simulink model "Cruise_Model_V8_QRTuning_TFLim"  (R2024a)
settings: Solver=ode23t  StartTime=0.0  StopTime=20  RelTol=1e-3
values from neighbouring files (symbols this model uses):
  F = fullfile(P,S(k).name)    [extractNACAdata.m]
  mission = struct()    [runMission.m]
  r = fuselage(i).diameter/2    [plotConfiguration.m]
  referenceGeo =     [alexisignoringme.mat]    (also in testing.mat)
undefined symbols (not defined in the file or in its folder): coefficients, dir, K, kb, kt, Light, MIL, Ue, Xe, Xes, xyz_tr
libraries: slpidlib x14, aerolibwind2 x8, aerolibatmos2 x4, shared6dof x1
(part 2 of 3)

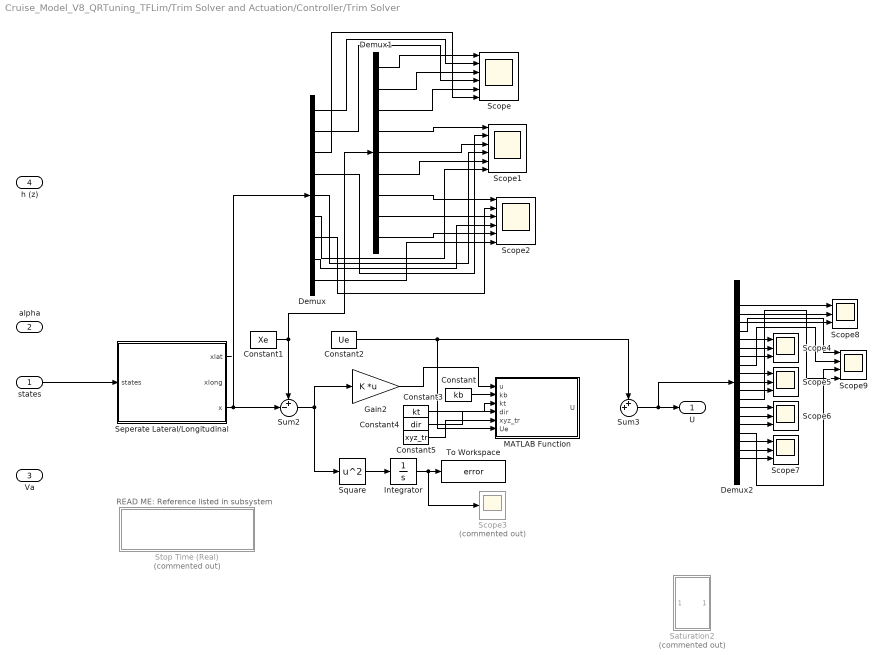
== system Cruise_Model_V8_QRTuning_TFLim/Trim Solver and Actuation/Controller/Trim Solver ==
  note: READ ME: Reference listed in subsystem
  states : Inport
  alpha : Inport  Port=2
  Va : Inport  Port=3
  h (z) : Inport  Port=4
  Constant : Constant  Value=kb
  Constant1 : Constant  Value=Xe
  Constant2 : Constant  Value=Ue
  Constant3 : Constant  Value=kt
  Constant4 : Constant  Value=dir
  Constant5 : Constant  Value=xyz_tr
  Demux : Demux  Outputs=9
  Demux1 : Demux  Outputs=9
  Demux2 : Demux  Outputs=19
  Gain2 : Gain  Gain=K  Multiplication=Matrix(K*u) (u vector)
  Integrator : Integrator
  MATLAB Function : MATLAB Function  TreatAsAtomicUnit=on
  Saturation2 : Subsystem  Commented=on
  Scope : Scope  NumInputPorts=6
  Scope1 : Scope  NumInputPorts=6
  Scope2 : Scope  NumInputPorts=6
  Scope3 : Scope  Commented=on
  Scope{4..8} (5 alike) : Scope  NumInputPorts=3
  Scope9 : Scope  NumInputPorts=4
  Seperate Lateral/Longitudinal : Subsystem
  Square : Math  Operator=square
  Stop Time (Real) : Subsystem  Commented=on
  Sum2 : Sum  Inputs=+-|
  Sum3 : Sum  Inputs=++|
  To Workspace : ToWorkspace  VariableName=error  SaveFormat=Timeseries  SampleTime=-1
  U : Outport
  wires:
  states/1 -> Seperate Lateral/Longitudinal/1(states)
  Seperate Lateral/Longitudinal/1(xlat) -> ?
  Seperate Lateral/Longitudinal/3(x) -> Demux/1, Sum2/2
  Constant2/1 -> Sum3/1, MATLAB Function/6(Ue)
  Constant1/1 -> Sum2/1, Demux1/1
  Square/1 -> Integrator/1
  Sum2/1 -> Square/1, Gain2/1
  Integrator/1 -> Scope3/1, To Workspace/1
  Demux1/1 -> Scope/1
  Demux/1 -> Scope/2
  Demux1/2 -> Scope/3
  Demux/2 -> Scope/4
  Demux1/3 -> Scope/5
  Demux/3 -> Scope/6
  Demux1/4 -> Scope1/1
  Demux1/5 -> Scope1/3
  Demux1/6 -> Scope1/5
  Demux/4 -> Scope1/2
  Demux/5 -> Scope1/4
  Demux/6 -> Scope1/6
  Demux1/7 -> Scope2/1
  Demux1/8 -> Scope2/3
  Demux1/9 -> Scope2/5
  Demux/7 -> Scope2/2
  Demux/8 -> Scope2/4
  Demux/9 -> Scope2/6
  Demux2/5 -> Scope4/1
  Demux2/6 -> Scope4/2
  Demux2/7 -> Scope4/3
  Demux2/9 -> Scope5/1
  Demux2/10 -> Scope5/2
  Demux2/11 -> Scope5/3
  Demux2/13 -> Scope6/1
  Demux2/14 -> Scope6/2
  Demux2/15 -> Scope6/3
  Demux2/17 -> Scope7/1
  Demux2/18 -> Scope7/2
  Demux2/19 -> Scope7/3
  Sum3/1 -> U/1, Demux2/1
  Gain2/1 -> MATLAB Function/1(u)
  Demux2/1 -> Scope8/1
  Demux2/2 -> Scope8/2
  Demux2/3 -> Scope8/3
  Demux2/4 -> Scope9/1
  Demux2/8 -> Scope9/2
  Demux2/12 -> Scope9/4
  Demux2/16 -> Scope9/3
  Constant/1 -> MATLAB Function/2(kb)
  Constant3/1 -> MATLAB Function/3(kt)
  Constant4/1 -> MATLAB Function/4(dir)
  Constant5/1 -> MATLAB Function/5(xyz_tr)

== system Cruise_Model_V8_QRTuning_TFLim/Atmospheric Effects/Atmospheric Effects1/Variant Subsystem/a ==
  h (z) : Inport
  Constant : Constant  Value=0
  ISA Atmosphere : aerolibatmos2/ISA Atmosphere Model  useExtended=off  action=Warning  custom=off  viscosityOut=off  g=9.80665  gamma=1.4  R=287.0531  L=0.0065  h_trop=11000  h_strat=20000  rho0=1.225  P0=101325  T0=288.15  h0=0  S=110.4  Tref=273.15  muref=1.716e-5
  Terminator1 : Terminator
  Terminator2 : Terminator
  Terminator3 : Terminator
  Air Density : Outport
  Vw : Outport  Port=2
  wires:
  h (z)/1 -> ISA Atmosphere/1
  ISA Atmosphere/2 -> Terminator1/1
  ISA Atmosphere/1 -> Terminator3/1
  ISA Atmosphere/4 -> Air Density/1
  ISA Atmosphere/3 -> Terminator2/1
  Constant/1 -> Vw/1

== system Cruise_Model_V8_QRTuning_TFLim/Atmospheric Effects/Atmospheric Effects1/Variant Subsystem/ag ==
  uvw_e : Inport
  h (z) : Inport  Port=2
  Demux : Demux  Outputs=3
  Discrete Wind Gust Model : aerolibwind2/Discrete Wind Gust Model  units=Metric (MKS)  Gx=on  Gy=on  Gz=on  t_0=40  d_m=[120 120 80]  v_m=[10 10 10]
  ISA Atmosphere : aerolibatmos2/ISA Atmosphere Model  useExtended=off  action=Warning  custom=off  viscosityOut=off  g=9.80665  gamma=1.4  R=287.0531  L=0.0065  h_trop=11000  h_strat=20000  rho0=1.225  P0=101325  T0=288.15  h0=0  S=110.4  Tref=273.15  muref=1.716e-5
  Terminator1 : Terminator
  Terminator2 : Terminator
  Terminator3 : Terminator
  Vw : Outport
  Air Density : Outport  Port=2
  wires:
  h (z)/1 -> ISA Atmosphere/1
  Demux/1 -> Discrete Wind Gust Model/1
  ISA Atmosphere/2 -> Terminator1/1
  ISA Atmosphere/1 -> Terminator3/1
  ISA Atmosphere/4 -> Air Density/1
  uvw_e/1 -> Demux/1
  ISA Atmosphere/3 -> Terminator2/1
  Discrete Wind Gust Model/1 -> Vw/1

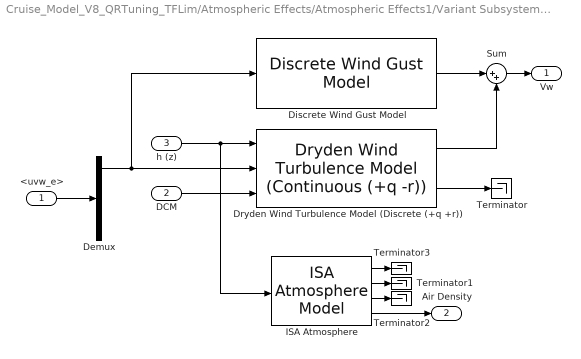
== system Cruise_Model_V8_QRTuning_TFLim/Atmospheric Effects/Atmospheric Effects1/Variant Subsystem/agt ==
  <uvw_e> : Inport
  DCM : Inport  Port=2
  h (z) : Inport  Port=3
  Demux : Demux  Outputs=3
  Discrete Wind Gust Model : aerolibwind2/Discrete Wind Gust Model  units=Metric (MKS)  Gx=on  Gy=on  Gz=on  t_0=40  d_m=[120 120 80]  v_m=[10 10 10]
  Dryden Wind Turbulence Model (Discrete (+q +r)) : aerolibwind2/Dryden Wind Turbulence Model  (Continuous (+q -r))  units=Metric (MKS)  spec=MIL-F-8785C  model=Continuous Dryden (+q -r)  W20=10  Wdeg=8  TurbProb=10^-2 - Light  L_high=533.4  Wingspan=7  ts=0.1  Seed=[23341 23342 23343 23344]  T_on=on
      settings: LibrarySourceBlock=|
      | aerolibwind2/Dryden Wind Turbulence Model
      | (Discrete (+q +r))
  ISA Atmosphere : aerolibatmos2/ISA Atmosphere Model  useExtended=off  action=Warning  custom=off  viscosityOut=off  g=9.80665  gamma=1.4  R=287.0531  L=0.0065  h_trop=11000  h_strat=20000  rho0=1.225  P0=101325  T0=288.15  h0=0  S=110.4  Tref=273.15  muref=1.716e-5
  Sum : Sum  Inputs=|++
  Terminator{,1..3} (4 alike) : Terminator
  Vw : Outport
  Air Density : Outport  Port=2
  wires:
  h (z)/1 -> Dryden Wind Turbulence Model (Discrete (+q +r))/1, ISA Atmosphere/1
  Demux/1 -> Dryden Wind Turbulence Model (Discrete (+q +r))/2, Discrete Wind Gust Model/1
  ISA Atmosphere/2 -> Terminator1/1
  ISA Atmosphere/1 -> Terminator3/1
  ISA Atmosphere/4 -> Air Density/1
  <uvw_e>/1 -> Demux/1
  DCM/1 -> Dryden Wind Turbulence Model (Discrete (+q +r))/3
  Dryden Wind Turbulence Model (Discrete (+q +r))/2 -> Terminator/1
  Sum/1 -> Vw/1
  ISA Atmosphere/3 -> Terminator2/1
  Dryden Wind Turbulence Model (Discrete (+q +r))/1 -> Sum/2
  Discrete Wind Gust Model/1 -> Sum/1

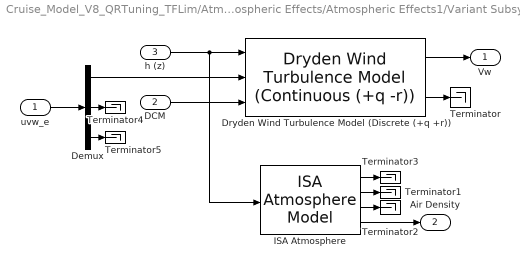
== system Cruise_Model_V8_QRTuning_TFLim/Atmospheric Effects/Atmospheric Effects1/Variant Subsystem/at ==
  uvw_e : Inport
  DCM : Inport  Port=2
  h (z) : Inport  Port=3
  Demux : Demux  Outputs=3
  Dryden Wind Turbulence Model (Discrete (+q +r)) : aerolibwind2/Dryden Wind Turbulence Model  (Continuous (+q -r))  units=Metric (MKS)  spec=MIL-F-8785C  model=Continuous Dryden (+q -r)  W20=10  Wdeg=8  TurbProb=10^-2 - Light  L_high=533.4  Wingspan=7  ts=0.1  Seed=[23341 23342 23343 23344]  T_on=on
      settings: LibrarySourceBlock=|
      | aerolibwind2/Dryden Wind Turbulence Model
      | (Discrete (+q +r))
  ISA Atmosphere : aerolibatmos2/ISA Atmosphere Model  useExtended=off  action=Warning  custom=off  viscosityOut=off  g=9.80665  gamma=1.4  R=287.0531  L=0.0065  h_trop=11000  h_strat=20000  rho0=1.225  P0=101325  T0=288.15  h0=0  S=110.4  Tref=273.15  muref=1.716e-5
  Terminator{,1..5} (6 alike) : Terminator
  Vw : Outport
  Air Density : Outport  Port=2
  wires:
  h (z)/1 -> Dryden Wind Turbulence Model (Discrete (+q +r))/1, ISA Atmosphere/1
  Demux/1 -> Dryden Wind Turbulence Model (Discrete (+q +r))/2
  ISA Atmosphere/2 -> Terminator1/1
  ISA Atmosphere/1 -> Terminator3/1
  ISA Atmosphere/4 -> Air Density/1
  uvw_e/1 -> Demux/1
  DCM/1 -> Dryden Wind Turbulence Model (Discrete (+q +r))/3
  Dryden Wind Turbulence Model (Discrete (+q +r))/2 -> Terminator/1
  ISA Atmosphere/3 -> Terminator2/1
  Demux/2 -> Terminator4/1
  Demux/3 -> Terminator5/1
  Dryden Wind Turbulence Model (Discrete (+q +r))/1 -> Vw/1

== system Cruise_Model_V8_QRTuning_TFLim/Atmospheric Effects/Atmospheric Effects1/Variant Subsystem/g ==
  uvw_e : Inport
  Constant : Constant  Value=1.225
  Demux : Demux  Outputs=3
  Discrete Wind Gust Model : aerolibwind2/Discrete Wind Gust Model  units=Metric (MKS)  Gx=on  Gy=on  Gz=on  t_0=40  d_m=[120 120 80]  v_m=[10 10 10]
  Vw : Outport
  Air Density : Outport  Port=2
  wires:
  Demux/1 -> Discrete Wind Gust Model/1
  uvw_e/1 -> Demux/1
  Discrete Wind Gust Model/1 -> Vw/1
  Constant/1 -> Air Density/1

== system Cruise_Model_V8_QRTuning_TFLim/Atmospheric Effects/Atmospheric Effects1/Variant Subsystem/gt ==
  <uvw_e> : Inport
  DCM : Inport  Port=2
  h (z) : Inport  Port=3
  Constant : Constant  Value=1.225
  Demux : Demux  Outputs=3
  Discrete Wind Gust Model : aerolibwind2/Discrete Wind Gust Model  units=Metric (MKS)  Gx=on  Gy=on  Gz=on  t_0=40  d_m=[120 120 80]  v_m=[10 10 10]
  Dryden Wind Turbulence Model (Discrete (+q +r)) : aerolibwind2/Dryden Wind Turbulence Model  (Continuous (+q -r))  units=Metric (MKS)  spec=MIL-F-8785C  model=Continuous Dryden (+q -r)  W20=10  Wdeg=8  TurbProb=10^-2 - Light  L_high=533.4  Wingspan=7  ts=0.1  Seed=[23341 23342 23343 23344]  T_on=on
      settings: LibrarySourceBlock=|
      | aerolibwind2/Dryden Wind Turbulence Model
      | (Discrete (+q +r))
  Sum : Sum  Inputs=|++
  Terminator : Terminator
  Vw : Outport
  Air Density : Outport  Port=2
  wires:
  h (z)/1 -> Dryden Wind Turbulence Model (Discrete (+q +r))/1
  Demux/1 -> Dryden Wind Turbulence Model (Discrete (+q +r))/2, Discrete Wind Gust Model/1
  <uvw_e>/1 -> Demux/1
  DCM/1 -> Dryden Wind Turbulence Model (Discrete (+q +r))/3
  Dryden Wind Turbulence Model (Discrete (+q +r))/2 -> Terminator/1
  Sum/1 -> Vw/1
  Dryden Wind Turbulence Model (Discrete (+q +r))/1 -> Sum/2
  Discrete Wind Gust Model/1 -> Sum/1
  Constant/1 -> Air Density/1

== system Cruise_Model_V8_QRTuning_TFLim/Atmospheric Effects/Atmospheric Effects1/Variant Subsystem/n ==
  Constant : Constant  Value=0
  Constant1 : Constant  Value=1.225
  Vw : Outport
  Air Density : Outport  Port=2
  wires:
  Constant/1 -> Vw/1
  Constant1/1 -> Air Density/1

== system Cruise_Model_V8_QRTuning_TFLim/Atmospheric Effects/Atmospheric Effects1/Variant Subsystem/t ==
  <uvw_e> : Inport
  DCM : Inport  Port=2
  h (z) : Inport  Port=3
  Constant1 : Constant  Value=1.225
  Demux : Demux  Outputs=3
  Dryden Wind Turbulence Model (Discrete (+q +r)) : aerolibwind2/Dryden Wind Turbulence Model  (Continuous (+q -r))  units=Metric (MKS)  spec=MIL-F-8785C  model=Continuous Dryden (+q -r)  W20=10  Wdeg=8  TurbProb=10^-2 - Light  L_high=533.4  Wingspan=7  ts=0.1  Seed=[23341 23342 23343 23344]  T_on=on
      settings: LibrarySourceBlock=|
      | aerolibwind2/Dryden Wind Turbulence Model
      | (Discrete (+q +r))
  Terminator : Terminator
  Vw : Outport
  Air Density : Outport  Port=2
  wires:
  h (z)/1 -> Dryden Wind Turbulence Model (Discrete (+q +r))/1
  Demux/1 -> Dryden Wind Turbulence Model (Discrete (+q +r))/2
  <uvw_e>/1 -> Demux/1
  DCM/1 -> Dryden Wind Turbulence Model (Discrete (+q +r))/3
  Dryden Wind Turbulence Model (Discrete (+q +r))/2 -> Terminator/1
  Constant1/1 -> Air Density/1
  Dryden Wind Turbulence Model (Discrete (+q +r))/1 -> Vw/1

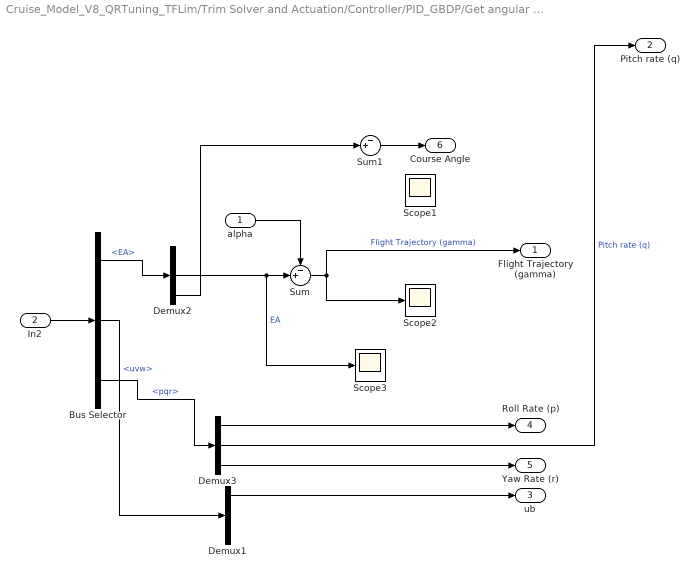
== system Cruise_Model_V8_QRTuning_TFLim/Trim Solver and Actuation/Controller/PID_GBDP/Get angular properties ==
  alpha : Inport
  In2 : Inport  Port=2
  Bus Selector : BusSelector  OutputSignals=EA,uvw,pqr
  Demux1 : Demux  Outputs=3
  Demux2 : Demux  Outputs=3
  Demux3 : Demux  Outputs=3
  Scope1 : Scope
  Scope2 : Scope
  Scope3 : Scope
  Sum : Sum  Inputs=-+|
  Sum1 : Sum  Inputs=-+|
  Flight Trajectory (gamma) : Outport
  Pitch rate (q) : Outport  Port=2
  ub : Outport  Port=3
  Roll Rate (p) : Outport  Port=4
  Yaw Rate (r) : Outport  Port=5
  Course Angle : Outport  Port=6
  wires:
  alpha/1 -> Sum/1
  Demux2/2 -> Sum/2, Scope3/1  "EA"
  Bus Selector/3 -> Demux3/1  "<pqr>"
  Sum/1 -> Flight Trajectory (gamma)/1, Scope2/1  "Flight Trajectory (gamma)"
  Bus Selector/1 -> Demux2/1  "<EA>"
  In2/1 -> Bus Selector/1
  Demux3/2 -> Pitch rate (q)/1  "Pitch rate (q)"
  Bus Selector/2 -> Demux1/1  "<uvw>"
  Demux1/1 -> ub/1
  Demux3/1 -> Roll Rate (p)/1
  Sum1/1 -> Course Angle/1
  Demux3/3 -> Yaw Rate (r)/1
  Demux2/3 -> Sum1/2

== system Cruise_Model_V8_QRTuning_TFLim/Trim Solver and Actuation/Controller/PID_GBDP/Step demand for testing ==
  In1 : Inport
  Mux1 : Mux  Inputs=2
  Scope2 : Scope
  Scope4 : Scope
  Step1 : Step  Time=60  Before=-500  After=-490  SampleTime=0
  Step2 : Step  Time=80  After=-10  SampleTime=0
  Step3 : Step  Time=120  After=20  SampleTime=0
  Step4 : Step  Time=120  After=20  SampleTime=0
  Sum : Sum  Inputs=++++
  To Workspace : ToWorkspace  VariableName=altitudeResponse  SaveFormat=Timeseries  SampleTime=-1
  Out1 : Outport
  wires:
  Step3/1 -> Sum/3
  Mux1/1 -> To Workspace/1, Scope4/1
  Sum/1 -> Out1/1, Mux1/1
  Step4/1 -> Sum/4
  Step1/1 -> Sum/1
  In1/1 -> Mux1/2, Scope2/1
  Step2/1 -> Sum/2

== system Cruise_Model_V8_QRTuning_TFLim/Trim Solver and Actuation/Controller/PID_GBDP/Step demand for testing1 ==
  Va : Inport
  Mux1 : Mux  Inputs=2
  Scope2 : Scope
  Scope4 : Scope
  Step1 : Step  Time=60  Before=25  After=31  SampleTime=0
  Step2 : Step  Time=80  After=-3  SampleTime=0
  Step3 : Step  Time=120  After=-5  SampleTime=0
  Step4 : Step  Time=100  After=8  SampleTime=0
  Step5 : Step  Time=140  After=-2  SampleTime=0
  Sum : Sum  Inputs=+++++
  To Workspace : ToWorkspace  VariableName=airspeedResponse  SaveFormat=Timeseries  SampleTime=-1
  Out1 : Outport
  wires:
  Step2/1 -> Sum/2
  Va/1 -> Scope2/1, Mux1/2
  Step1/1 -> Sum/1
  Step4/1 -> Sum/4
  Sum/1 -> Mux1/1, Out1/1
  Mux1/1 -> Scope4/1, To Workspace/1
  Step3/1 -> Sum/3
  Step5/1 -> Sum/5

== system Cruise_Model_V8_QRTuning_TFLim/Trim Solver and Actuation/Controller/PID_GBDP/Step demand for testing2 ==
  Va : Inport
  Mux1 : Mux  Inputs=2
  Scope2 : Scope
  Scope4 : Scope
  Step1 : Step  Time=60  Before=0.1  After=0.2  SampleTime=0
  Step2 : Step  Time=80  After=-0.4  SampleTime=0
  Step3 : Step  Time=120  After=-0.2  SampleTime=0
  Step4 : Step  Time=100  After=0.6  SampleTime=0
  Step5 : Step  Time=140  After=-0.4  SampleTime=0
  Sum : Sum  Inputs=+++++
  To Workspace : ToWorkspace  VariableName=headingAngleResponse  SaveFormat=Timeseries  SampleTime=-1
  Out1 : Outport
  wires:
  Step5/1 -> Sum/5
  Step3/1 -> Sum/3
  Mux1/1 -> To Workspace/1, Scope4/1
  Sum/1 -> Out1/1, Mux1/1
  Step4/1 -> Sum/4
  Step1/1 -> Sum/1
  Va/1 -> Mux1/2, Scope2/1
  Step2/1 -> Sum/2

== system Cruise_Model_V8_QRTuning_TFLim/Trim Solver and Actuation/Controller/PID_GBDP_withThrust/Altitude Control Path ==
  note: Altitude Control Path
  h (z) : Inport
  Flight Trajectory : Inport  Port=2
  Pitch Rate : Inport  Port=3
  Demand : Inport  Port=4
  PID Controller10 : slpidlib/PID Controller  Controller=PID  Form=Parallel  TimeDomain=Continuous-time  UseExternalTs=off  SampleTime=-1  IntegratorMethod=Forward Euler  FilterMethod=Forward Euler  ControllerParametersSource=internal  P=-0.89713711901533  I=-27.659938076894  UseKiTs=off  D=-0.00302643608728309  UseExternalDerivativeSource=off  N=142.832860389355  UseFilter=on  TunerSelectOption=Transfer Function Based (PID Tuner App)  InitialConditionSource=internal  InitialConditionForIntegrator=0.44  InitialConditionForFilter=0  DifferentiatorICPrevScaledInput=0  ExternalReset=none  TrackingMode=off  Kt=1  LimitOutput=on  SatLimitsSource=internal  UpperSaturationLimit=0.44  LowerSaturationLimit=-0.44  LinearizeAsGain=on  AntiWindupMode=clamping  Kb=1  LimitIntegrator=off  UpperIntegratorSaturationLimit=inf  LowerIntegratorSaturationLimit=-inf  POutMin=[]  POutMax=[]  IOutMin=[]  IOutMax=[]  DOutMin=[]  DOutMax=[]  NOutMin=[]  NOutMax=[]  SumOutMin=[]  SumOutMax=[]  SaturationOutMin=[]  SaturationOutMax=[]  PParamMin=[]  PParamMax=[]  IParamMin=[]  IParamMax=[]  DParamMin=[]  DParamMax=[]  NParamMin=[]  NParamMax=[]  KbParamMin=[]  KbParamMax=[]  KtParamMin=[]  KtParamMax=[]  KbOutMin=[]  KbOutMax=[]  KtOutMin=[]  KtOutMax=[]  IntegratorOutMin=[]  IntegratorOutMax=[]  FilterOutMin=[]  FilterOutMax=[]  SumI1OutMin=[]  SumI1OutMax=[]  SumI2OutMin=[]  SumI2OutMax=[]  SumI3OutMin=[]  SumI3OutMax=[]  SumI4OutMin=[]  SumI4OutMax=[]  SumDOutMin=[]  SumDOutMax=[]  DifferentiatorOutMin=[]  DifferentiatorOutMax=[]  FilterDiffOutCoefMin=[]  FilterDiffOutCoefMax=[]  ReciprocalOutMin=[]  ReciprocalOutMax=[]  SumDenOutMin=[]  SumDenOutMax=[]  SumNumOutMin=[]  SumNumOutMax=[]  DivideOutMin=[]  DivideOutMax=[]  UdiffTsProdOutMin=[]  UdiffTsProdOutMax=[]  NTsProdOutMin=[]  NTsProdOutMax=[]  UintegralTsProdOutMin=[]  UintegralTsProdOutMax=[]  UngainTsProdOutMin=[]  UngainTsProdOutMax=[]  ClampingZeroOutDataTypeStr=Inherit: Inherit via back propagation  ClampingZeroOutMin=[]  ClampingZeroOutMax=[]  FilterDenConstantOutDataTypeStr=Inherit: Inherit via back propagation  FilterDenConstantOutMin=[]  FilterDenConstantOutMax=[]  PCopyOutDataTypeStr=Inherit: Inherit via back propagation  PCopyOutMin=[]  PCopyOutMax=[]  NCopyOutDataTypeStr=Inherit: Inherit via back propagation  NCopyOutMin=[]  NCopyOutMax=[]  IntegratorContinuousStateAttributes=''  IntegratorStateMustResolveToSignalObject=off  IntegratorRTWStateStorageClass=Auto  FilterContinuousStateAttributes=''  FilterStateMustResolveToSignalObject=off  FilterRTWStateStorageClass=Auto  ParallelPVariant=InternalParameters  IdealPVariant=Disabled  IVariant=InternalParameters  DVariant=InternalParameters  IntegratorVariant=Continuous  SatVariant=Enabled  AWVariant=ContClampingParallel  PCopyVariant=Disabled  TRVariant=Disabled  FdbkBlocksVariant=Forward  IdealPFdbkVariant=Disabled  SatFdbkVariant=Disabled  DerivativeFilterVariant=ContFilter  NVariant=InternalParameters  NCopyVariant=Disabled  FilterICVariant=InternalICsFilter  IntegratorICVariant=InternalICs  ExternalResetVariant=Disabled  TRSumVariant=Passthrough  SumFdbkVariant=Disabled  SumVariant=Sum_PID  TsampFilterVariant=InternalTs  TsampNgainVariant=Passthrough  TsampIntegralVariant=Disabled_SignalSpec  ExternalSaturationOutDataTypeStr=Inherit: Same as second input  DerivativeSourceVariant=ErrorSignal
  PID Controller4 : slpidlib/PID Controller  Controller=PID  Form=Parallel  TimeDomain=Continuous-time  UseExternalTs=off  SampleTime=-1  IntegratorMethod=Forward Euler  FilterMethod=Forward Euler  ControllerParametersSource=internal  P=-0.487630187489664  I=-0.0704619791070383  UseKiTs=off  D=-0.813392530162756  UseExternalDerivativeSource=off  N=7.99704030727873  UseFilter=on  TunerSelectOption=Transfer Function Based (PID Tuner App)  InitialConditionSource=internal  InitialConditionForIntegrator=0.1  InitialConditionForFilter=0  DifferentiatorICPrevScaledInput=0  ExternalReset=none  TrackingMode=off  Kt=1  LimitOutput=on  SatLimitsSource=internal  UpperSaturationLimit=0.44  LowerSaturationLimit=-0.44  LinearizeAsGain=on  AntiWindupMode=clamping  Kb=1  LimitIntegrator=off  UpperIntegratorSaturationLimit=inf  LowerIntegratorSaturationLimit=-inf  POutMin=[]  POutMax=[]  IOutMin=[]  IOutMax=[]  DOutMin=[]  DOutMax=[]  NOutMin=[]  NOutMax=[]  SumOutMin=[]  SumOutMax=[]  SaturationOutMin=[]  SaturationOutMax=[]  PParamMin=[]  PParamMax=[]  IParamMin=[]  IParamMax=[]  DParamMin=[]  DParamMax=[]  NParamMin=[]  NParamMax=[]  KbParamMin=[]  KbParamMax=[]  KtParamMin=[]  KtParamMax=[]  KbOutMin=[]  KbOutMax=[]  KtOutMin=[]  KtOutMax=[]  IntegratorOutMin=[]  IntegratorOutMax=[]  FilterOutMin=[]  FilterOutMax=[]  SumI1OutMin=[]  SumI1OutMax=[]  SumI2OutMin=[]  SumI2OutMax=[]  SumI3OutMin=[]  SumI3OutMax=[]  SumI4OutMin=[]  SumI4OutMax=[]  SumDOutMin=[]  SumDOutMax=[]  DifferentiatorOutMin=[]  DifferentiatorOutMax=[]  FilterDiffOutCoefMin=[]  FilterDiffOutCoefMax=[]  ReciprocalOutMin=[]  ReciprocalOutMax=[]  SumDenOutMin=[]  SumDenOutMax=[]  SumNumOutMin=[]  SumNumOutMax=[]  DivideOutMin=[]  DivideOutMax=[]  UdiffTsProdOutMin=[]  UdiffTsProdOutMax=[]  NTsProdOutMin=[]  NTsProdOutMax=[]  UintegralTsProdOutMin=[]  UintegralTsProdOutMax=[]  UngainTsProdOutMin=[]  UngainTsProdOutMax=[]  ClampingZeroOutDataTypeStr=Inherit: Inherit via back propagation  ClampingZeroOutMin=[]  ClampingZeroOutMax=[]  FilterDenConstantOutDataTypeStr=Inherit: Inherit via back propagation  FilterDenConstantOutMin=[]  FilterDenConstantOutMax=[]  PCopyOutDataTypeStr=Inherit: Inherit via back propagation  PCopyOutMin=[]  PCopyOutMax=[]  NCopyOutDataTypeStr=Inherit: Inherit via back propagation  NCopyOutMin=[]  NCopyOutMax=[]  IntegratorContinuousStateAttributes=''  IntegratorStateMustResolveToSignalObject=off  IntegratorRTWStateStorageClass=Auto  FilterContinuousStateAttributes=''  FilterStateMustResolveToSignalObject=off  FilterRTWStateStorageClass=Auto  ParallelPVariant=InternalParameters  IdealPVariant=Disabled  IVariant=InternalParameters  DVariant=InternalParameters  IntegratorVariant=Continuous  SatVariant=Enabled  AWVariant=ContClampingParallel  PCopyVariant=Disabled  TRVariant=Disabled  FdbkBlocksVariant=Forward  IdealPFdbkVariant=Disabled  SatFdbkVariant=Disabled  DerivativeFilterVariant=ContFilter  NVariant=InternalParameters  NCopyVariant=Disabled  FilterICVariant=InternalICsFilter  IntegratorICVariant=InternalICs  ExternalResetVariant=Disabled  TRSumVariant=Passthrough  SumFdbkVariant=Disabled  SumVariant=Sum_PID  TsampFilterVariant=InternalTs  TsampNgainVariant=Passthrough  TsampIntegralVariant=Disabled_SignalSpec  ExternalSaturationOutDataTypeStr=Inherit: Same as second input  DerivativeSourceVariant=ErrorSignal
  PID Controller9 : slpidlib/PID Controller  Controller=PID  Form=Parallel  TimeDomain=Continuous-time  UseExternalTs=off  SampleTime=-1  IntegratorMethod=Forward Euler  FilterMethod=Forward Euler  ControllerParametersSource=internal  P=0.0886412010406481  I=0.0145723289748373  UseKiTs=off  D=0.129850691124493  UseExternalDerivativeSource=off  N=8.9831666478447  UseFilter=on  TunerSelectOption=Transfer Function Based (PID Tuner App)  InitialConditionSource=internal  InitialConditionForIntegrator=0  InitialConditionForFilter=0  DifferentiatorICPrevScaledInput=0  ExternalReset=none  TrackingMode=off  Kt=1  LimitOutput=on  SatLimitsSource=internal  UpperSaturationLimit=0.09  LowerSaturationLimit=-0.3  LinearizeAsGain=off  AntiWindupMode=clamping  Kb=1  LimitIntegrator=off  UpperIntegratorSaturationLimit=inf  LowerIntegratorSaturationLimit=-inf  POutMin=[]  POutMax=[]  IOutMin=[]  IOutMax=[]  DOutMin=[]  DOutMax=[]  NOutMin=[]  NOutMax=[]  SumOutMin=[]  SumOutMax=[]  SaturationOutMin=[]  SaturationOutMax=[]  PParamMin=[]  PParamMax=[]  IParamMin=[]  IParamMax=[]  DParamMin=[]  DParamMax=[]  NParamMin=[]  NParamMax=[]  KbParamMin=[]  KbParamMax=[]  KtParamMin=[]  KtParamMax=[]  KbOutMin=[]  KbOutMax=[]  KtOutMin=[]  KtOutMax=[]  IntegratorOutMin=[]  IntegratorOutMax=[]  FilterOutMin=[]  FilterOutMax=[]  SumI1OutMin=[]  SumI1OutMax=[]  SumI2OutMin=[]  SumI2OutMax=[]  SumI3OutMin=[]  SumI3OutMax=[]  SumI4OutMin=[]  SumI4OutMax=[]  SumDOutMin=[]  SumDOutMax=[]  DifferentiatorOutMin=[]  DifferentiatorOutMax=[]  FilterDiffOutCoefMin=[]  FilterDiffOutCoefMax=[]  ReciprocalOutMin=[]  ReciprocalOutMax=[]  SumDenOutMin=[]  SumDenOutMax=[]  SumNumOutMin=[]  SumNumOutMax=[]  DivideOutMin=[]  DivideOutMax=[]  UdiffTsProdOutMin=[]  UdiffTsProdOutMax=[]  NTsProdOutMin=[]  NTsProdOutMax=[]  UintegralTsProdOutMin=[]  UintegralTsProdOutMax=[]  UngainTsProdOutMin=[]  UngainTsProdOutMax=[]  ClampingZeroOutDataTypeStr=Inherit: Inherit via back propagation  ClampingZeroOutMin=[]  ClampingZeroOutMax=[]  FilterDenConstantOutDataTypeStr=Inherit: Inherit via back propagation  FilterDenConstantOutMin=[]  FilterDenConstantOutMax=[]  PCopyOutDataTypeStr=Inherit: Inherit via back propagation  PCopyOutMin=[]  PCopyOutMax=[]  NCopyOutDataTypeStr=Inherit: Inherit via back propagation  NCopyOutMin=[]  NCopyOutMax=[]  IntegratorContinuousStateAttributes=''  IntegratorStateMustResolveToSignalObject=off  IntegratorRTWStateStorageClass=Auto  FilterContinuousStateAttributes=''  FilterStateMustResolveToSignalObject=off  FilterRTWStateStorageClass=Auto  ParallelPVariant=InternalParameters  IdealPVariant=Disabled  IVariant=InternalParameters  DVariant=InternalParameters  IntegratorVariant=Continuous  SatVariant=Enabled  AWVariant=ContClampingParallel  PCopyVariant=Disabled  TRVariant=Disabled  FdbkBlocksVariant=Forward  IdealPFdbkVariant=Disabled  SatFdbkVariant=Disabled  DerivativeFilterVariant=ContFilter  NVariant=InternalParameters  NCopyVariant=Disabled  FilterICVariant=InternalICsFilter  IntegratorICVariant=InternalICs  ExternalResetVariant=Disabled  TRSumVariant=Passthrough  SumFdbkVariant=Disabled  SumVariant=Sum_PID  TsampFilterVariant=InternalTs  TsampNgainVariant=Passthrough  TsampIntegralVariant=Disabled_SignalSpec  ExternalSaturationOutDataTypeStr=Inherit: Same as second input  DerivativeSourceVariant=ErrorSignal
  Step demand for testing : Subsystem
  Subtract : Sum  Inputs=|-+
  Subtract1 : Sum  Inputs=|+-
  Subtract3 : Sum  Inputs=|-+
  dE : Outport
  wires:
  PID Controller9/1 -> Subtract/1
  h (z)/1 -> Step demand for testing/1(In1), Subtract1/1
  Subtract/1 -> PID Controller4/1
  Pitch Rate/1 -> Subtract3/2
  Subtract1/1 -> PID Controller9/1
  Subtract3/1 -> PID Controller10/1
  PID Controller4/1 -> Subtract3/1
  Flight Trajectory/1 -> Subtract/2
  PID Controller10/1 -> dE/1
  Demand/1 -> Subtract1/2

== system Cruise_Model_V8_QRTuning_TFLim/Trim Solver and Actuation/Controller/PID_GBDP_withThrust/Course Angle Control Path ==
  note: Course Angle Control Path
  Course Angle : Inport
  In2 : Inport  Port=2
  PID Controller2 : slpidlib/PID Controller  Controller=PID  Form=Parallel  TimeDomain=Continuous-time  UseExternalTs=off  SampleTime=-1  IntegratorMethod=Forward Euler  FilterMethod=Forward Euler  ControllerParametersSource=internal  P=0.61259661356046  I=0.000997427544306601  UseKiTs=off  D=0.894500555152138  UseExternalDerivativeSource=off  N=62.5354170285902  UseFilter=on  TunerSelectOption=Transfer Function Based (PID Tuner App)  InitialConditionSource=internal  InitialConditionForIntegrator=0  InitialConditionForFilter=0  DifferentiatorICPrevScaledInput=0  ExternalReset=none  TrackingMode=off  Kt=1  LimitOutput=on  SatLimitsSource=internal  UpperSaturationLimit=0.52  LowerSaturationLimit=-0.52  LinearizeAsGain=on  AntiWindupMode=clamping  Kb=1  LimitIntegrator=off  UpperIntegratorSaturationLimit=inf  LowerIntegratorSaturationLimit=-inf  POutMin=[]  POutMax=[]  IOutMin=[]  IOutMax=[]  DOutMin=[]  DOutMax=[]  NOutMin=[]  NOutMax=[]  SumOutMin=[]  SumOutMax=[]  SaturationOutMin=[]  SaturationOutMax=[]  PParamMin=[]  PParamMax=[]  IParamMin=[]  IParamMax=[]  DParamMin=[]  DParamMax=[]  NParamMin=[]  NParamMax=[]  KbParamMin=[]  KbParamMax=[]  KtParamMin=[]  KtParamMax=[]  KbOutMin=[]  KbOutMax=[]  KtOutMin=[]  KtOutMax=[]  IntegratorOutMin=[]  IntegratorOutMax=[]  FilterOutMin=[]  FilterOutMax=[]  SumI1OutMin=[]  SumI1OutMax=[]  SumI2OutMin=[]  SumI2OutMax=[]  SumI3OutMin=[]  SumI3OutMax=[]  SumI4OutMin=[]  SumI4OutMax=[]  SumDOutMin=[]  SumDOutMax=[]  DifferentiatorOutMin=[]  DifferentiatorOutMax=[]  FilterDiffOutCoefMin=[]  FilterDiffOutCoefMax=[]  ReciprocalOutMin=[]  ReciprocalOutMax=[]  SumDenOutMin=[]  SumDenOutMax=[]  SumNumOutMin=[]  SumNumOutMax=[]  DivideOutMin=[]  DivideOutMax=[]  UdiffTsProdOutMin=[]  UdiffTsProdOutMax=[]  NTsProdOutMin=[]  NTsProdOutMax=[]  UintegralTsProdOutMin=[]  UintegralTsProdOutMax=[]  UngainTsProdOutMin=[]  UngainTsProdOutMax=[]  ClampingZeroOutDataTypeStr=Inherit: Inherit via back propagation  ClampingZeroOutMin=[]  ClampingZeroOutMax=[]  FilterDenConstantOutDataTypeStr=Inherit: Inherit via back propagation  FilterDenConstantOutMin=[]  FilterDenConstantOutMax=[]  PCopyOutDataTypeStr=Inherit: Inherit via back propagation  PCopyOutMin=[]  PCopyOutMax=[]  NCopyOutDataTypeStr=Inherit: Inherit via back propagation  NCopyOutMin=[]  NCopyOutMax=[]  IntegratorContinuousStateAttributes=''  IntegratorStateMustResolveToSignalObject=off  IntegratorRTWStateStorageClass=Auto  FilterContinuousStateAttributes=''  FilterStateMustResolveToSignalObject=off  FilterRTWStateStorageClass=Auto  ParallelPVariant=InternalParameters  IdealPVariant=Disabled  IVariant=InternalParameters  DVariant=InternalParameters  IntegratorVariant=Continuous  SatVariant=Enabled  AWVariant=ContClampingParallel  PCopyVariant=Disabled  TRVariant=Disabled  FdbkBlocksVariant=Forward  IdealPFdbkVariant=Disabled  SatFdbkVariant=Disabled  DerivativeFilterVariant=ContFilter  NVariant=InternalParameters  NCopyVariant=Disabled  FilterICVariant=InternalICsFilter  IntegratorICVariant=InternalICs  ExternalResetVariant=Disabled  TRSumVariant=Passthrough  SumFdbkVariant=Disabled  SumVariant=Sum_PID  TsampFilterVariant=InternalTs  TsampNgainVariant=Passthrough  TsampIntegralVariant=Disabled_SignalSpec  ExternalSaturationOutDataTypeStr=Inherit: Same as second input  DerivativeSourceVariant=ErrorSignal
  PID Controller7 : slpidlib/PID Controller  Controller=PID  Form=Parallel  TimeDomain=Continuous-time  UseExternalTs=off  SampleTime=-1  IntegratorMethod=Forward Euler  FilterMethod=Forward Euler  ControllerParametersSource=internal  P=0.013462751880451  I=6.03710934436948e-04  UseKiTs=off  D=0.667051880736134  UseExternalDerivativeSource=off  N=87.8445721553921  UseFilter=on  TunerSelectOption=Transfer Function Based (PID Tuner App)  InitialConditionSource=internal  InitialConditionForIntegrator=0  InitialConditionForFilter=0  DifferentiatorICPrevScaledInput=0  ExternalReset=none  TrackingMode=off  Kt=1  LimitOutput=on  SatLimitsSource=internal  UpperSaturationLimit=0.52  LowerSaturationLimit=-0.52  LinearizeAsGain=on  AntiWindupMode=none  Kb=1  LimitIntegrator=off  UpperIntegratorSaturationLimit=inf  LowerIntegratorSaturationLimit=-inf  POutMin=[]  POutMax=[]  IOutMin=[]  IOutMax=[]  DOutMin=[]  DOutMax=[]  NOutMin=[]  NOutMax=[]  SumOutMin=[]  SumOutMax=[]  SaturationOutMin=[]  SaturationOutMax=[]  PParamMin=[]  PParamMax=[]  IParamMin=[]  IParamMax=[]  DParamMin=[]  DParamMax=[]  NParamMin=[]  NParamMax=[]  KbParamMin=[]  KbParamMax=[]  KtParamMin=[]  KtParamMax=[]  KbOutMin=[]  KbOutMax=[]  KtOutMin=[]  KtOutMax=[]  IntegratorOutMin=[]  IntegratorOutMax=[]  FilterOutMin=[]  FilterOutMax=[]  SumI1OutMin=[]  SumI1OutMax=[]  SumI2OutMin=[]  SumI2OutMax=[]  SumI3OutMin=[]  SumI3OutMax=[]  SumI4OutMin=[]  SumI4OutMax=[]  SumDOutMin=[]  SumDOutMax=[]  DifferentiatorOutMin=[]  DifferentiatorOutMax=[]  FilterDiffOutCoefMin=[]  FilterDiffOutCoefMax=[]  ReciprocalOutMin=[]  ReciprocalOutMax=[]  SumDenOutMin=[]  SumDenOutMax=[]  SumNumOutMin=[]  SumNumOutMax=[]  DivideOutMin=[]  DivideOutMax=[]  UdiffTsProdOutMin=[]  UdiffTsProdOutMax=[]  NTsProdOutMin=[]  NTsProdOutMax=[]  UintegralTsProdOutMin=[]  UintegralTsProdOutMax=[]  UngainTsProdOutMin=[]  UngainTsProdOutMax=[]  ClampingZeroOutDataTypeStr=Inherit: Inherit via back propagation  ClampingZeroOutMin=[]  ClampingZeroOutMax=[]  FilterDenConstantOutDataTypeStr=Inherit: Inherit via back propagation  FilterDenConstantOutMin=[]  FilterDenConstantOutMax=[]  PCopyOutDataTypeStr=Inherit: Inherit via back propagation  PCopyOutMin=[]  PCopyOutMax=[]  NCopyOutDataTypeStr=Inherit: Inherit via back propagation  NCopyOutMin=[]  NCopyOutMax=[]  IntegratorContinuousStateAttributes=''  IntegratorStateMustResolveToSignalObject=off  IntegratorRTWStateStorageClass=Auto  FilterContinuousStateAttributes=''  FilterStateMustResolveToSignalObject=off  FilterRTWStateStorageClass=Auto  ParallelPVariant=InternalParameters  IdealPVariant=Disabled  IVariant=InternalParameters  DVariant=InternalParameters  IntegratorVariant=Continuous  SatVariant=Enabled  AWVariant=Passthrough  PCopyVariant=Disabled  TRVariant=Disabled  FdbkBlocksVariant=Forward  IdealPFdbkVariant=Disabled  SatFdbkVariant=Disabled  DerivativeFilterVariant=ContFilter  NVariant=InternalParameters  NCopyVariant=Disabled  FilterICVariant=InternalICsFilter  IntegratorICVariant=InternalICs  ExternalResetVariant=Disabled  TRSumVariant=Passthrough  SumFdbkVariant=Disabled  SumVariant=Sum_PID  TsampFilterVariant=InternalTs  TsampNgainVariant=Passthrough  TsampIntegralVariant=Disabled_SignalSpec  ExternalSaturationOutDataTypeStr=Inherit: Same as second input  DerivativeSourceVariant=ErrorSignal
  Step demand for testing2 : Subsystem
  Subtract2 : Sum  Inputs=|+-
  dA : Outport
  dR : Outport  Port=2
  wires:
  Subtract2/1 -> PID Controller2/1, PID Controller7/1
  Course Angle/1 -> Step demand for testing2/1(Va), Subtract2/1
  PID Controller7/1 -> dA/1
  PID Controller2/1 -> dR/1
  In2/1 -> Subtract2/2

== system Cruise_Model_V8_QRTuning_TFLim/Trim Solver and Actuation/Controller/PID_GBDP_withThrust/Get angular properties ==
  alpha : Inport
  In2 : Inport  Port=2
  Bus Selector : BusSelector  OutputSignals=EA,uvw,pqr
  Demux1 : Demux  Outputs=3
  Demux2 : Demux  Outputs=3
  Demux3 : Demux  Outputs=3
  Sum : Sum  Inputs=-+|
  Flight Trajectory (gamma) : Outport
  Pitch rate (q) : Outport  Port=2
  ub : Outport  Port=3
  Roll Rate (p) : Outport  Port=4
  Yaw Rate (r) : Outport  Port=5
  Course Angle : Outport  Port=6
  wires:
  alpha/1 -> Sum/1
  Demux2/2 -> Sum/2  "EA"
  Bus Selector/3 -> Demux3/1  "<pqr>"
  Sum/1 -> Flight Trajectory (gamma)/1  "Flight Trajectory (gamma)"
  Bus Selector/1 -> Demux2/1  "<EA>"
  In2/1 -> Bus Selector/1
  Demux3/2 -> Pitch rate (q)/1  "Pitch rate (q)"
  Bus Selector/2 -> Demux1/1  "<uvw>"
  Demux1/1 -> ub/1
  Demux3/1 -> Roll Rate (p)/1
  Demux2/3 -> Course Angle/1
  Demux3/3 -> Yaw Rate (r)/1

== system Cruise_Model_V8_QRTuning_TFLim/Trim Solver and Actuation/Controller/PID_GBDP_withThrust/Subsystem ==
  note: Airspeed Control Path
  Va : Inport
  Demand : Inport  Port=2
  PID Controller1 : slpidlib/PID Controller  Controller=PID  Form=Parallel  TimeDomain=Continuous-time  UseExternalTs=off  SampleTime=-1  IntegratorMethod=Forward Euler  FilterMethod=Forward Euler  ControllerParametersSource=internal  P=-124.171962714531  I=-8.86566238209981  UseKiTs=off  D=35.5117343437496  UseExternalDerivativeSource=off  N=0.73276571825447  UseFilter=on  TunerSelectOption=Transfer Function Based (PID Tuner App)  InitialConditionSource=internal  InitialConditionForIntegrator=0  InitialConditionForFilter=1  DifferentiatorICPrevScaledInput=0  ExternalReset=none  TrackingMode=off  Kt=1  LimitOutput=on  SatLimitsSource=internal  UpperSaturationLimit=300  LowerSaturationLimit=0  LinearizeAsGain=on  AntiWindupMode=clamping  Kb=1  LimitIntegrator=off  UpperIntegratorSaturationLimit=inf  LowerIntegratorSaturationLimit=-inf  POutMin=[]  POutMax=[]  IOutMin=[]  IOutMax=[]  DOutMin=[]  DOutMax=[]  NOutMin=[]  NOutMax=[]  SumOutMin=[]  SumOutMax=[]  SaturationOutMin=[]  SaturationOutMax=[]  PParamMin=[]  PParamMax=[]  IParamMin=[]  IParamMax=[]  DParamMin=[]  DParamMax=[]  NParamMin=[]  NParamMax=[]  KbParamMin=[]  KbParamMax=[]  KtParamMin=[]  KtParamMax=[]  KbOutMin=[]  KbOutMax=[]  KtOutMin=[]  KtOutMax=[]  IntegratorOutMin=[]  IntegratorOutMax=[]  FilterOutMin=[]  FilterOutMax=[]  SumI1OutMin=[]  SumI1OutMax=[]  SumI2OutMin=[]  SumI2OutMax=[]  SumI3OutMin=[]  SumI3OutMax=[]  SumI4OutMin=[]  SumI4OutMax=[]  SumDOutMin=[]  SumDOutMax=[]  DifferentiatorOutMin=[]  DifferentiatorOutMax=[]  FilterDiffOutCoefMin=[]  FilterDiffOutCoefMax=[]  ReciprocalOutMin=[]  ReciprocalOutMax=[]  SumDenOutMin=[]  SumDenOutMax=[]  SumNumOutMin=[]  SumNumOutMax=[]  DivideOutMin=[]  DivideOutMax=[]  UdiffTsProdOutMin=[]  UdiffTsProdOutMax=[]  NTsProdOutMin=[]  NTsProdOutMax=[]  UintegralTsProdOutMin=[]  UintegralTsProdOutMax=[]  UngainTsProdOutMin=[]  UngainTsProdOutMax=[]  ClampingZeroOutDataTypeStr=Inherit: Inherit via back propagation  ClampingZeroOutMin=[]  ClampingZeroOutMax=[]  FilterDenConstantOutDataTypeStr=Inherit: Inherit via back propagation  FilterDenConstantOutMin=[]  FilterDenConstantOutMax=[]  PCopyOutDataTypeStr=Inherit: Inherit via back propagation  PCopyOutMin=[]  PCopyOutMax=[]  NCopyOutDataTypeStr=Inherit: Inherit via back propagation  NCopyOutMin=[]  NCopyOutMax=[]  IntegratorContinuousStateAttributes=''  IntegratorStateMustResolveToSignalObject=off  IntegratorRTWStateStorageClass=Auto  FilterContinuousStateAttributes=''  FilterStateMustResolveToSignalObject=off  FilterRTWStateStorageClass=Auto  ParallelPVariant=InternalParameters  IdealPVariant=Disabled  IVariant=InternalParameters  DVariant=InternalParameters  IntegratorVariant=Continuous  SatVariant=Enabled  AWVariant=ContClampingParallel  PCopyVariant=Disabled  TRVariant=Disabled  FdbkBlocksVariant=Forward  IdealPFdbkVariant=Disabled  SatFdbkVariant=Disabled  DerivativeFilterVariant=ContFilter  NVariant=InternalParameters  NCopyVariant=Disabled  FilterICVariant=InternalICsFilter  IntegratorICVariant=InternalICs  ExternalResetVariant=Disabled  TRSumVariant=Passthrough  SumFdbkVariant=Disabled  SumVariant=Sum_PID  TsampFilterVariant=InternalTs  TsampNgainVariant=Passthrough  TsampIntegralVariant=Disabled_SignalSpec  ExternalSaturationOutDataTypeStr=Inherit: Same as second input  DerivativeSourceVariant=ErrorSignal
  Step demand for testing1 : Subsystem
  Subtract5 : Sum  Inputs=|+-
  dT : Outport
  wires:
  PID Controller1/1 -> dT/1
  Subtract5/1 -> PID Controller1/1
  Va/1 -> Subtract5/1, Step demand for testing1/1(Va)
  Demand/1 -> Subtract5/2
  Step demand for testing1/1(Out1) -> ?

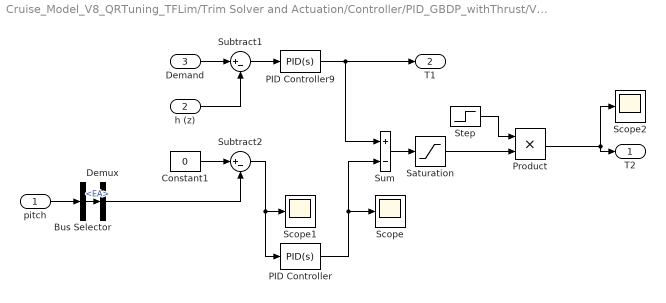
== system Cruise_Model_V8_QRTuning_TFLim/Trim Solver and Actuation/Controller/PID_GBDP_withThrust/VTOL Control Path ==
  pitch : Inport
  h (z) : Inport  Port=2
  Demand : Inport  Port=3
  Bus Selector : BusSelector  OutputSignals=EA
  Constant1 : Constant  Value=0
  Demux : Demux  Outputs=3
  PID Controller : slpidlib/PID Controller  Controller=PID  Form=Parallel  TimeDomain=Continuous-time  UseExternalTs=off  SampleTime=-1  IntegratorMethod=Forward Euler  FilterMethod=Forward Euler  ControllerParametersSource=internal  P=2347  I=2604  UseKiTs=off  D=519  UseExternalDerivativeSource=off  N=129  UseFilter=on  TunerSelectOption=Transfer Function Based (PID Tuner App)  InitialConditionSource=internal  InitialConditionForIntegrator=0  InitialConditionForFilter=0  DifferentiatorICPrevScaledInput=0  ExternalReset=none  TrackingMode=off  Kt=1  LimitOutput=on  SatLimitsSource=internal  UpperSaturationLimit=800  LowerSaturationLimit=-800  LinearizeAsGain=on  AntiWindupMode=clamping  Kb=1  LimitIntegrator=off  UpperIntegratorSaturationLimit=inf  LowerIntegratorSaturationLimit=-inf  POutMin=[]  POutMax=[]  IOutMin=[]  IOutMax=[]  DOutMin=[]  DOutMax=[]  NOutMin=[]  NOutMax=[]  SumOutMin=[]  SumOutMax=[]  SaturationOutMin=[]  SaturationOutMax=[]  PParamMin=[]  PParamMax=[]  IParamMin=[]  IParamMax=[]  DParamMin=[]  DParamMax=[]  NParamMin=[]  NParamMax=[]  KbParamMin=[]  KbParamMax=[]  KtParamMin=[]  KtParamMax=[]  KbOutMin=[]  KbOutMax=[]  KtOutMin=[]  KtOutMax=[]  IntegratorOutMin=[]  IntegratorOutMax=[]  FilterOutMin=[]  FilterOutMax=[]  SumI1OutMin=[]  SumI1OutMax=[]  SumI2OutMin=[]  SumI2OutMax=[]  SumI3OutMin=[]  SumI3OutMax=[]  SumI4OutMin=[]  SumI4OutMax=[]  SumDOutMin=[]  SumDOutMax=[]  DifferentiatorOutMin=[]  DifferentiatorOutMax=[]  FilterDiffOutCoefMin=[]  FilterDiffOutCoefMax=[]  ReciprocalOutMin=[]  ReciprocalOutMax=[]  SumDenOutMin=[]  SumDenOutMax=[]  SumNumOutMin=[]  SumNumOutMax=[]  DivideOutMin=[]  DivideOutMax=[]  UdiffTsProdOutMin=[]  UdiffTsProdOutMax=[]  NTsProdOutMin=[]  NTsProdOutMax=[]  UintegralTsProdOutMin=[]  UintegralTsProdOutMax=[]  UngainTsProdOutMin=[]  UngainTsProdOutMax=[]  ClampingZeroOutDataTypeStr=Inherit: Inherit via back propagation  ClampingZeroOutMin=[]  ClampingZeroOutMax=[]  FilterDenConstantOutDataTypeStr=Inherit: Inherit via back propagation  FilterDenConstantOutMin=[]  FilterDenConstantOutMax=[]  PCopyOutDataTypeStr=Inherit: Inherit via back propagation  PCopyOutMin=[]  PCopyOutMax=[]  NCopyOutDataTypeStr=Inherit: Inherit via back propagation  NCopyOutMin=[]  NCopyOutMax=[]  IntegratorContinuousStateAttributes=''  IntegratorStateMustResolveToSignalObject=off  IntegratorRTWStateStorageClass=Auto  FilterContinuousStateAttributes=''  FilterStateMustResolveToSignalObject=off  FilterRTWStateStorageClass=Auto  ParallelPVariant=InternalParameters  IdealPVariant=Disabled  IVariant=InternalParameters  DVariant=InternalParameters  IntegratorVariant=Continuous  SatVariant=Enabled  AWVariant=ContClampingParallel  PCopyVariant=Disabled  TRVariant=Disabled  FdbkBlocksVariant=Forward  IdealPFdbkVariant=Disabled  SatFdbkVariant=Disabled  DerivativeFilterVariant=ContFilter  NVariant=InternalParameters  NCopyVariant=Disabled  FilterICVariant=InternalICsFilter  IntegratorICVariant=InternalICs  ExternalResetVariant=Disabled  TRSumVariant=Passthrough  SumFdbkVariant=Disabled  SumVariant=Sum_PID  TsampFilterVariant=InternalTs  TsampNgainVariant=Passthrough  TsampIntegralVariant=Disabled_SignalSpec  ExternalSaturationOutDataTypeStr=Inherit: Same as second input  DerivativeSourceVariant=ErrorSignal
  PID Controller9 : slpidlib/PID Controller  Controller=PID  Form=Parallel  TimeDomain=Continuous-time  UseExternalTs=off  SampleTime=-1  IntegratorMethod=Forward Euler  FilterMethod=Forward Euler  ControllerParametersSource=internal  P=-174.901958260333  I=-41.0371926298995  UseKiTs=off  D=-183.043785953636  UseExternalDerivativeSource=off  N=27.3346026399604  UseFilter=on  TunerSelectOption=Transfer Function Based (PID Tuner App)  InitialConditionSource=internal  InitialConditionForIntegrator=0  InitialConditionForFilter=0  DifferentiatorICPrevScaledInput=0  ExternalReset=none  TrackingMode=off  Kt=1  LimitOutput=on  SatLimitsSource=internal  UpperSaturationLimit=2000  LowerSaturationLimit=0  LinearizeAsGain=off  AntiWindupMode=clamping  Kb=1  LimitIntegrator=off  UpperIntegratorSaturationLimit=inf  LowerIntegratorSaturationLimit=-inf  POutMin=[]  POutMax=[]  IOutMin=[]  IOutMax=[]  DOutMin=[]  DOutMax=[]  NOutMin=[]  NOutMax=[]  SumOutMin=[]  SumOutMax=[]  SaturationOutMin=[]  SaturationOutMax=[]  PParamMin=[]  PParamMax=[]  IParamMin=[]  IParamMax=[]  DParamMin=[]  DParamMax=[]  NParamMin=[]  NParamMax=[]  KbParamMin=[]  KbParamMax=[]  KtParamMin=[]  KtParamMax=[]  KbOutMin=[]  KbOutMax=[]  KtOutMin=[]  KtOutMax=[]  IntegratorOutMin=[]  IntegratorOutMax=[]  FilterOutMin=[]  FilterOutMax=[]  SumI1OutMin=[]  SumI1OutMax=[]  SumI2OutMin=[]  SumI2OutMax=[]  SumI3OutMin=[]  SumI3OutMax=[]  SumI4OutMin=[]  SumI4OutMax=[]  SumDOutMin=[]  SumDOutMax=[]  DifferentiatorOutMin=[]  DifferentiatorOutMax=[]  FilterDiffOutCoefMin=[]  FilterDiffOutCoefMax=[]  ReciprocalOutMin=[]  ReciprocalOutMax=[]  SumDenOutMin=[]  SumDenOutMax=[]  SumNumOutMin=[]  SumNumOutMax=[]  DivideOutMin=[]  DivideOutMax=[]  UdiffTsProdOutMin=[]  UdiffTsProdOutMax=[]  NTsProdOutMin=[]  NTsProdOutMax=[]  UintegralTsProdOutMin=[]  UintegralTsProdOutMax=[]  UngainTsProdOutMin=[]  UngainTsProdOutMax=[]  ClampingZeroOutDataTypeStr=Inherit: Inherit via back propagation  ClampingZeroOutMin=[]  ClampingZeroOutMax=[]  FilterDenConstantOutDataTypeStr=Inherit: Inherit via back propagation  FilterDenConstantOutMin=[]  FilterDenConstantOutMax=[]  PCopyOutDataTypeStr=Inherit: Inherit via back propagation  PCopyOutMin=[]  PCopyOutMax=[]  NCopyOutDataTypeStr=Inherit: Inherit via back propagation  NCopyOutMin=[]  NCopyOutMax=[]  IntegratorContinuousStateAttributes=''  IntegratorStateMustResolveToSignalObject=off  IntegratorRTWStateStorageClass=Auto  FilterContinuousStateAttributes=''  FilterStateMustResolveToSignalObject=off  FilterRTWStateStorageClass=Auto  ParallelPVariant=InternalParameters  IdealPVariant=Disabled  IVariant=InternalParameters  DVariant=InternalParameters  IntegratorVariant=Continuous  SatVariant=Enabled  AWVariant=ContClampingParallel  PCopyVariant=Disabled  TRVariant=Disabled  FdbkBlocksVariant=Forward  IdealPFdbkVariant=Disabled  SatFdbkVariant=Disabled  DerivativeFilterVariant=ContFilter  NVariant=InternalParameters  NCopyVariant=Disabled  FilterICVariant=InternalICsFilter  IntegratorICVariant=InternalICs  ExternalResetVariant=Disabled  TRSumVariant=Passthrough  SumFdbkVariant=Disabled  SumVariant=Sum_PID  TsampFilterVariant=InternalTs  TsampNgainVariant=Passthrough  TsampIntegralVariant=Disabled_SignalSpec  ExternalSaturationOutDataTypeStr=Inherit: Same as second input  DerivativeSourceVariant=ErrorSignal
  Product : Product
  Saturation : Saturate  UpperLimit=9000  LowerLimit=0
  Scope : Scope
  Scope1 : Scope
  Scope2 : Scope
  Step : Step  Time=max(mission.trans.t)  Before=1  After=0  SampleTime=0
  Subtract1 : Sum  Inputs=|+-
  Subtract2 : Sum  Inputs=|+-
  Sum : Sum  Inputs=+-
  T2 : Outport
  T1 : Outport  Port=2
  wires:
  Demand/1 -> Subtract1/1
  h (z)/1 -> Subtract1/2
  Subtract1/1 -> PID Controller9/1
  Constant1/1 -> Subtract2/1
  pitch/1 -> Bus Selector/1
  Subtract2/1 -> PID Controller/1, Scope1/1
  PID Controller9/1 -> Sum/1, T1/1
  Sum/1 -> Saturation/1
  PID Controller/1 -> Sum/2, Scope/1
  Bus Selector/1 -> Demux/1  "<EA>"
  Demux/2 -> Subtract2/2
  Product/1 -> T2/1, Scope2/1
  Saturation/1 -> Product/2
  Step/1 -> Product/1

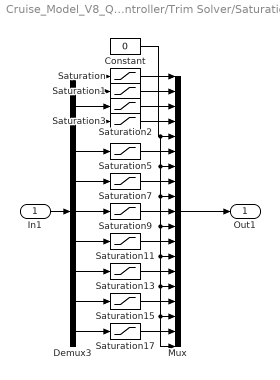
== system Cruise_Model_V8_QRTuning_TFLim/Trim Solver and Actuation/Controller/Trim Solver/Saturation2 ==
  In1 : Inport
  Constant : Constant  Value=0
  Demux3 : Demux  Outputs=19
  Mux : Mux  Inputs=19
  Saturation : Saturate  UpperLimit=0.55  LowerLimit=-0.55
  Saturation1 : Saturate  UpperLimit=0.55  LowerLimit=-0.55
  Saturation{3,7,11,15} (4 alike) : Saturate  UpperLimit=6e3  LowerLimit=0
  Saturation{5,9,13,17} (4 alike) : Saturate  UpperLimit=0.01  LowerLimit=-0.01
  Saturation2 : Saturate  UpperLimit=0.55  LowerLimit=-0.55
  Out1 : Outport
  wires:
  Constant/1 -> Mux/5, Mux/7, Mux/9, Mux/11, Mux/13, Mux/15, Mux/17, Mux/19
  Demux3/2 -> Saturation1/1
  Demux3/4 -> Saturation3/1
  Demux3/14 -> Saturation13/1
  Saturation3/1 -> Mux/4
  Saturation11/1 -> Mux/12
  Saturation5/1 -> Mux/6
  Demux3/10 -> Saturation9/1
  Saturation9/1 -> Mux/10
  Saturation15/1 -> Mux/16
  Demux3/1 -> Saturation/1
  Demux3/8 -> Saturation7/1
  Demux3/18 -> Saturation17/1
  In1/1 -> Demux3/1
  Saturation1/1 -> Mux/2
  Demux3/3 -> Saturation2/1
  Saturation7/1 -> Mux/8
  Demux3/6 -> Saturation5/1
  Saturation/1 -> Mux/1
  Saturation13/1 -> Mux/14
  Demux3/16 -> Saturation15/1
  Saturation17/1 -> Mux/18
  Saturation2/1 -> Mux/3
  Demux3/12 -> Saturation11/1
  Mux/1 -> Out1/1

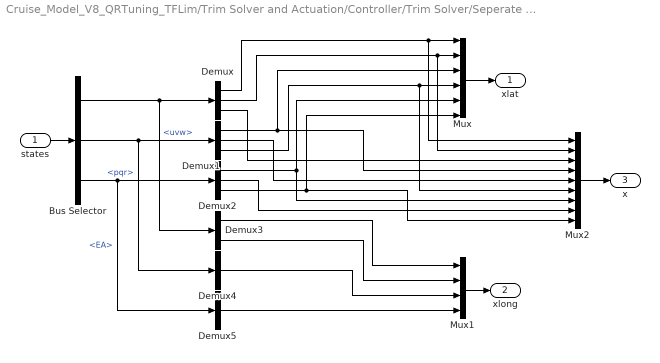
== system Cruise_Model_V8_QRTuning_TFLim/Trim Solver and Actuation/Controller/Trim Solver/Seperate Lateral//Longitudinal ==
  states : Inport
  Bus Selector : BusSelector  OutputSignals=uvw,pqr,EA
  Demux{,1..5} (6 alike) : Demux  Outputs=3
  Mux : Mux  Inputs=6
  Mux1 : Mux
  Mux2 : Mux  Inputs=9
  xlat : Outport
  xlong : Outport  Port=2
  x : Outport  Port=3
  wires:
  states/1 -> Bus Selector/1
  Mux/1 -> xlat/1
  Mux1/1 -> xlong/1
  Bus Selector/1 -> Demux/1, Demux3/1  "<uvw>"
  Bus Selector/2 -> Demux1/1, Demux4/1  "<pqr>"
  Bus Selector/3 -> Demux5/1, Demux2/1  "<EA>"
  Demux/1 -> Mux2/1, Mux/1
  Demux/2 -> Mux2/2, Mux/2
  Demux1/1 -> Mux2/4, Mux/3
  Demux1/3 -> Mux2/6, Mux/4
  Demux2/1 -> Mux2/7, Mux/5
  Demux2/3 -> Mux2/9, Mux/6
  Demux3/1 -> Mux1/1
  Demux3/3 -> Mux1/2
  Demux4/2 -> Mux1/3
  Demux5/2 -> Mux1/4
  Mux2/1 -> x/1
  Demux/3 -> Mux2/3
  Demux1/2 -> Mux2/5
  Demux2/2 -> Mux2/8

== system Cruise_Model_V8_QRTuning_TFLim/Trim Solver and Actuation/Controller/Trim Solver/Stop Time (Real) ==
  note: Source: Phillippe Martin (2016)
  note: https://www.researchgate.net/post/How-can-I-put-the-REAL-elapsed-time-as-a-constraint-in-a-Simulink-simulation
  Constant : Constant
  Display : Display  Commented=on
  MATLAB Function : MATLAB Function  TreatAsAtomicUnit=on
  Relational Operator : RelationalOperator  OutDataTypeStr=boolean  InputSameDT=off
  Stop Simulation : Stop
  wires:
  Constant/1 -> Relational Operator/2
  Relational Operator/1 -> Stop Simulation/1
  MATLAB Function/1(y) -> Display/1, Relational Operator/1

== system Cruise_Model_V8_QRTuning_TFLim/Trim Solver and Actuation/Controller/PID_GBDP_withThrust/Altitude Control Path/Step demand for testing ==
  In1 : Inport
  Mux1 : Mux  Inputs=2
  Scope2 : Scope
  Scope4 : Scope
  Step1 : Step  Time=60  Before=-500  After=-490  SampleTime=0
  Step2 : Step  Time=80  After=-10  SampleTime=0
  Step3 : Step  Time=120  After=20  SampleTime=0
  Step4 : Step  Time=120  After=20  SampleTime=0
  Sum : Sum  Inputs=++++
  To Workspace : ToWorkspace  VariableName=altitudeResponse  SaveFormat=Timeseries  SampleTime=-1
  Out1 : Outport
  wires:
  Step3/1 -> Sum/3
  Mux1/1 -> To Workspace/1, Scope4/1
  Sum/1 -> Out1/1, Mux1/1
  Step4/1 -> Sum/4
  Step1/1 -> Sum/1
  In1/1 -> Mux1/2, Scope2/1
  Step2/1 -> Sum/2

== system Cruise_Model_V8_QRTuning_TFLim/Trim Solver and Actuation/Controller/PID_GBDP_withThrust/Course Angle Control Path/Step demand for testing2 ==
  Va : Inport
  Mux1 : Mux  Inputs=2
  Scope2 : Scope
  Scope4 : Scope
  Step1 : Step  Time=60  Before=0.1  After=0.2  SampleTime=0
  Step2 : Step  Time=80  After=-0.4  SampleTime=0
  Step3 : Step  Time=120  After=-0.2  SampleTime=0
  Step4 : Step  Time=100  After=0.6  SampleTime=0
  Step5 : Step  Time=140  After=-0.4  SampleTime=0
  Sum : Sum  Inputs=+++++
  To Workspace : ToWorkspace  VariableName=headingAngleResponse  SaveFormat=Timeseries  SampleTime=-1
  Out1 : Outport
  wires:
  Step5/1 -> Sum/5
  Step3/1 -> Sum/3
  Mux1/1 -> To Workspace/1, Scope4/1
  Sum/1 -> Out1/1, Mux1/1
  Step4/1 -> Sum/4
  Step1/1 -> Sum/1
  Va/1 -> Mux1/2, Scope2/1
  Step2/1 -> Sum/2
